simulink model "RST_CU_ESTIMATOR"  (R2018a)
settings: Solver=VariableStepAuto  StartTime=0.0  StopTime=100  RelTol=1e-3
values from neighbouring files (symbols this model uses):
  a22 = -2*beta*(c+f10)/numitor    (= -0.0723201373103)    [Proiect_script_IRA2.m]    (also in decupalre.m; trying.m)
  a23 = -M*g*L*f10/numitor    (= -43.7694067093)    [Proiect_script_IRA2.m]    (also in decupalre.m; trying.m)
  a24 = 2*beta*(c+f10)/numitor    (= 0.0723201373103)    [Proiect_script_IRA2.m]    (also in decupalre.m; trying.m)
  a42 = 2*beta*(d+f10)/numitor    (= 0.0279773616358)    [Proiect_script_IRA2.m]    (also in decupalre.m; trying.m)
  a43 = d*M*g*L/numitor    (= 43.7747367103)    [Proiect_script_IRA2.m]    (also in decupalre.m; trying.m)
  a44 = 2*beta*(d+f10)/numitor    (= 0.0279773616358)    [Proiect_script_IRA2.m]    (also in decupalre.m = -0.0279773616358; trying.m = -0.0279773616358)
  a66 = ((-W*W*beta)/(2*R*R))/(m*W*W/2+W*W/(2*R*R)*(Jw+Jm)+Jphi)    (= -0.112438053457)    [Proiect_script_IRA2.m]    (also in decupalre.m; trying.m)
  b21 = alfa*(c+f10)/numitor    (= 1.04508868945)    [Proiect_script_IRA2.m]    (also in decupalre.m; trying.m)
  b22 = alfa*(c+f10)/numitor    (= 1.04508868945)    [Proiect_script_IRA2.m]    (also in decupalre.m; trying.m)
  b41 = -alfa*(d+f10)/numitor    (= -0.404297133465)    [Proiect_script_IRA2.m]    (also in decupalre.m; trying.m)
  b42 = -alfa*(d+f10)/numitor    (= -0.404297133465)    [Proiect_script_IRA2.m]    (also in decupalre.m; trying.m)
  b61 = ((-W*alfa)/(2*R))/(m*W*W/2+W*W/(2*R*R)*(Jw+Jm)+Jphi)    (= -0.609310260785)    [Proiect_script_IRA2.m]    (also in decupalre.m; trying.m)
  b62 = ((-W*alfa)/(2*R))/(m*W*W/2+W*W/(2*R*R)*(Jw+Jm)+Jphi)    (= -0.609310260785)    [Proiect_script_IRA2.m]    (also in decupalre.m; trying.m)
  F1 = inv(C1/(-A0)*B1)    [Proiect_script_IRA2.m]    (also in decupalre.m; trying.m)
  k1 = acker(A1,B1,[-50 -50 -50 -50])    [Proiect_script_IRA2.m]    (also in decupalre.m = acker(A1,B1,[-10 -10 -10 -10]); trying.m = acker(A1,B1,[-2 -2 -2 -2]))
  k3 = acker(A2,B2,[-50 -50])    [Proiect_script_IRA2.m]    (also in decupalre.m = acker(A2,B2,[-1 -1]); trying.m = acker(A2,B2,[-0.01 -0.01]))
  Lt1 = acker(A1',C1',[-1000 -1000 -1000 -1000])    [Proiect_script_IRA2.m]    (also in trying.m)
  Lt3 = acker(A2',C2',[-1000 -1000])    [Proiect_script_IRA2.m]    (also in trying.m)
settings Model: Creator=Andrei  LastModifiedBy=Andrei

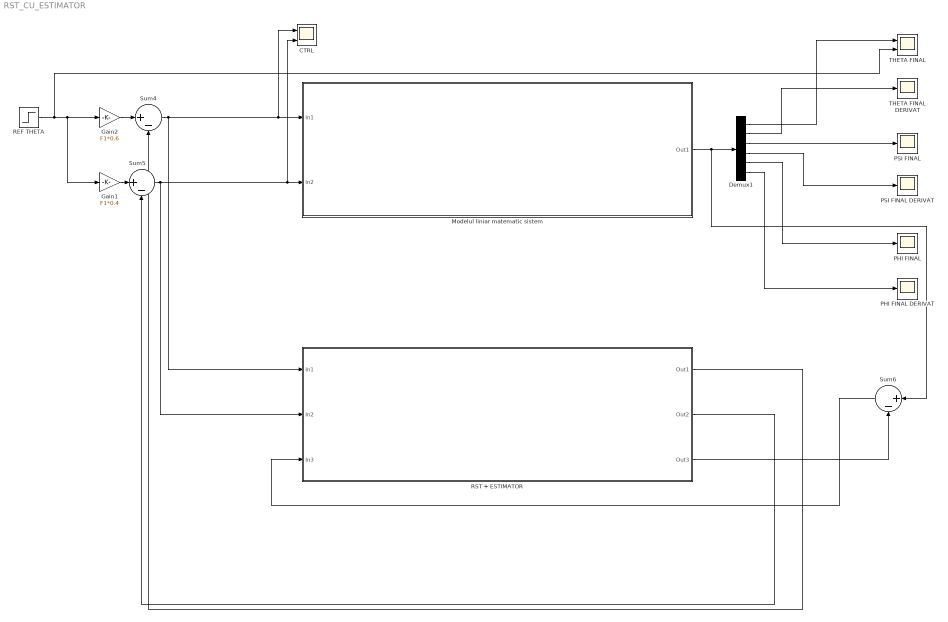
== system RST_CU_ESTIMATOR ==
  "CTRL " : Scope  NumInputPorts=2
  Demux1 : Demux  Outputs=6
  Gain1 : Gain  Gain=F1*0.4
  Gain2 : Gain  Gain=F1*0.6
  Modelul liniar matematic sistem : Subsystem
  PHI FINAL : Scope
  "PHI FINAL DERIVAT " : Scope
  PSI FINAL : Scope
  "PSI FINAL DERIVAT " : Scope
  "REF THETA " : Step  SampleTime=0
  "RST + ESTIMATOR " : Subsystem
  Sum4 : Sum  Inputs=|+-
  Sum5 : Sum  Inputs=|+-
  Sum6 : Sum  Inputs=|+-
  THETA FINAL : Scope  NumInputPorts=2
  "THETA FINAL DERIVAT " : Scope
  wires:
  Demux1/4 -> "PSI FINAL DERIVAT "/1
  "RST + ESTIMATOR "/1(Out1) -> Sum4/2
  Demux1/3 -> PSI FINAL/1
  Demux1/6 -> "PHI FINAL DERIVAT "/1
  Demux1/5 -> PHI FINAL/1
  Sum5/1 -> "RST + ESTIMATOR "/2(In2), Modelul liniar matematic sistem/2(In2), "CTRL "/2
  "RST + ESTIMATOR "/3(Out3) -> Sum6/2
  Demux1/1 -> THETA FINAL/1
  Gain2/1 -> Sum4/1
  Sum4/1 -> "RST + ESTIMATOR "/1(In1), Modelul liniar matematic sistem/1(In1), "CTRL "/1
  "RST + ESTIMATOR "/2(Out2) -> Sum5/2
  Modelul liniar matematic sistem/1(Out1) -> Demux1/1, Sum6/1
  Demux1/2 -> "THETA FINAL DERIVAT "/1
  Sum6/1 -> "RST + ESTIMATOR "/3(In3)
  "REF THETA "/1 -> THETA FINAL/2, Gain1/1, Gain2/1
  Gain1/1 -> Sum5/1

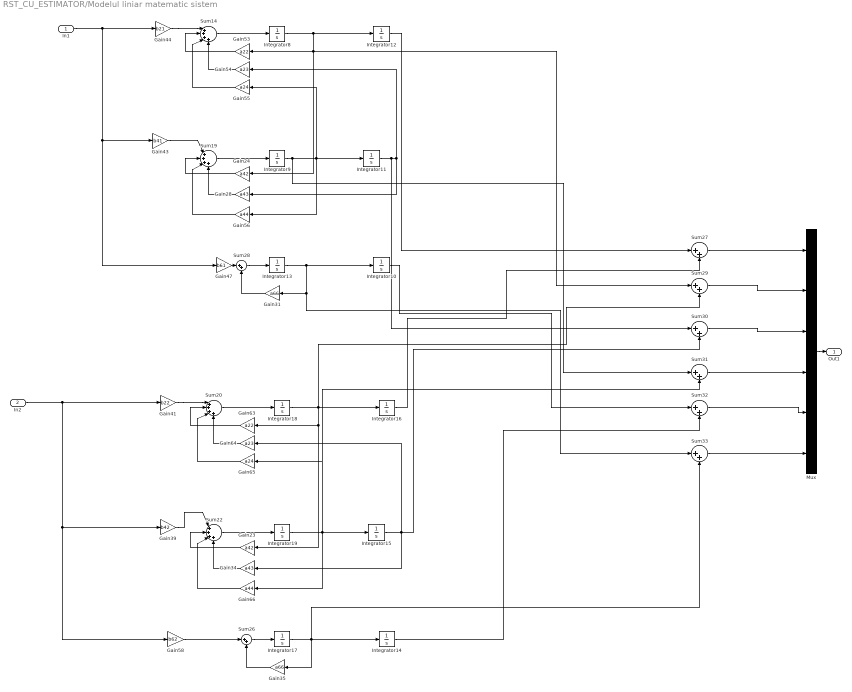
== system RST_CU_ESTIMATOR/Modelul liniar matematic sistem ==
  In1 : Inport
  In2 : Inport  Port=2
  Gain23 : Gain  Gain=a42
  Gain24 : Gain  Gain=a42
  Gain28 : Gain  Gain=a43
  Gain31 : Gain  Gain=a66
  Gain34 : Gain  Gain=a43
  Gain35 : Gain  Gain=a66
  Gain39 : Gain  Gain=b42
  Gain41 : Gain  Gain=b22
  Gain43 : Gain  Gain=b41
  Gain44 : Gain  Gain=b21
  Gain47 : Gain  Gain=b61
  Gain53 : Gain  Gain=a22
  Gain54 : Gain  Gain=a23
  Gain55 : Gain  Gain=a24
  Gain56 : Gain  Gain=a44
  Gain58 : Gain  Gain=b62
  Gain63 : Gain  Gain=a22
  Gain64 : Gain  Gain=a23
  Gain65 : Gain  Gain=a24
  Gain66 : Gain  Gain=a44
  Integrator{8..19} (12 alike) : Integrator
  Mux : Mux  Inputs=6
  Sum{14,19..20,22} (4 alike) : Sum  Inputs=|++++
  Sum{26..33} (8 alike) : Sum  Inputs=|++
  Out1 : Outport
  wires:
  In2/1 -> Gain41/1, Gain58/1, Gain39/1
  In1/1 -> Gain44/1, Gain43/1, Gain47/1
  Gain58/1 -> Sum26/1
  Sum26/1 -> Integrator17/1
  Integrator10/1 -> Sum32/1
  Gain56/1 -> Sum19/3
  Gain65/1 -> Sum20/3
  Integrator12/1 -> Sum27/1
  Sum29/1 -> Mux/2
  Sum31/1 -> Mux/4
  Gain23/1 -> Sum22/2
  Gain63/1 -> Sum20/2
  Gain35/1 -> Sum26/2
  Gain43/1 -> Sum19/1
  Sum28/1 -> Integrator13/1
  Gain47/1 -> Sum28/1
  Gain28/1 -> Sum19/4
  Integrator15/1 -> Gain34/1, Gain64/1, Sum30/2
  Integrator16/1 -> Sum27/2
  Sum27/1 -> Mux/1
  Gain34/1 -> Sum22/4
  Gain41/1 -> Sum20/1
  Integrator13/1 -> Integrator10/1, Gain31/1, Sum33/1
  Integrator11/1 -> Gain28/1, Gain54/1, Sum30/1
  Gain54/1 -> Sum14/4
  Integrator14/1 -> Sum32/2
  Gain64/1 -> Sum20/4
  Sum33/1 -> Mux/6
  Sum19/1 -> Integrator9/1
  Gain53/1 -> Sum14/2
  Gain24/1 -> Sum19/2
  Integrator18/1 -> Integrator16/1, Gain63/1, Gain23/1, Sum29/2
  Mux/1 -> Out1/1
  Sum22/1 -> Integrator19/1
  Integrator8/1 -> Integrator12/1, Gain53/1, Sum29/1, Gain24/1
  Gain44/1 -> Sum14/1
  Sum30/1 -> Mux/3
  Integrator17/1 -> Sum33/2, Integrator14/1, Gain35/1
  Sum14/1 -> Integrator8/1
  Sum20/1 -> Integrator18/1
  Gain55/1 -> Sum14/3
  Gain39/1 -> Sum22/1
  Sum32/1 -> Mux/5
  Integrator19/1 -> Gain65/1, Gain66/1, Sum31/2, Integrator15/1
  Gain66/1 -> Sum22/3
  Gain31/1 -> Sum28/2
  Integrator9/1 -> Integrator11/1, Gain55/1, Gain56/1, Sum31/1

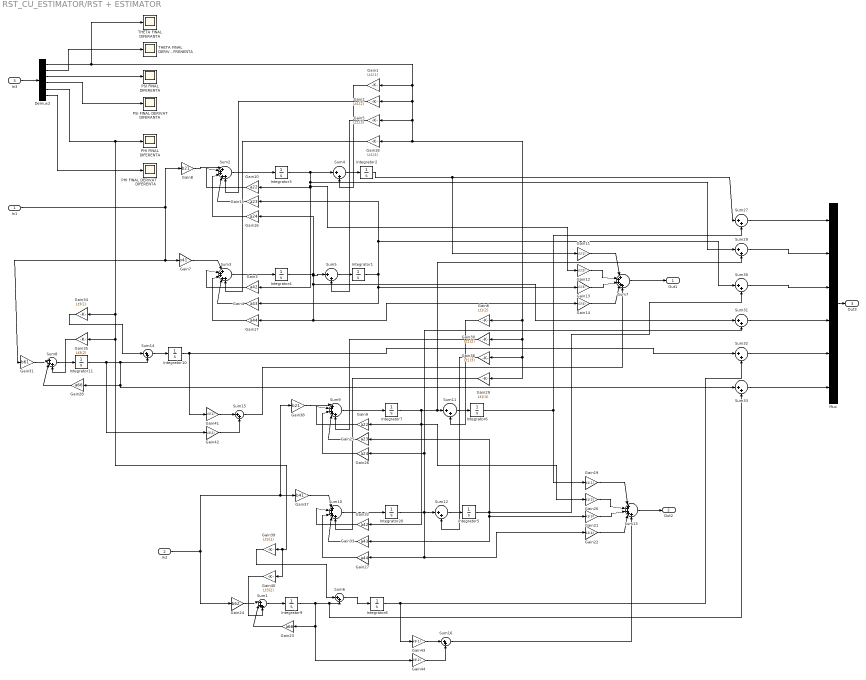
== system RST_CU_ESTIMATOR/RST + ESTIMATOR  ==
  In1 : Inport
  In2 : Inport  Port=2
  In3 : Inport  Port=3
  Demux2 : Demux  Outputs=6
  Gain1 : Gain  Gain=Lt1(1)
  Gain10 : Gain  Gain=a22
  Gain11 : Gain  Gain=k1(1)
  Gain12 : Gain  Gain=k1(2)
  Gain13 : Gain  Gain=k1(3)
  Gain14 : Gain  Gain=k1(4)
  Gain15 : Gain  Gain=a23
  Gain16 : Gain  Gain=a24
  Gain17 : Gain  Gain=a44
  Gain18 : Gain  Gain=Lt1(4)
  Gain19 : Gain  Gain=k1(1)
  Gain2 : Gain  Gain=Lt1(2)
  Gain20 : Gain  Gain=k1(2)
  Gain21 : Gain  Gain=k1(3)
  Gain22 : Gain  Gain=k1(4)
  Gain23 : Gain  Gain=a66
  Gain24 : Gain  Gain=b62
  Gain25 : Gain  Gain=a23
  Gain26 : Gain  Gain=a24
  Gain27 : Gain  Gain=a44
  Gain28 : Gain  Gain=a66
  Gain29 : Gain  Gain=Lt1(4)
  Gain3 : Gain  Gain=a42
  Gain30 : Gain  Gain=Lt1(2)
  Gain31 : Gain  Gain=b61
  Gain32 : Gain  Gain=a42
  Gain33 : Gain  Gain=a43
  Gain34 : Gain  Gain=Lt3(1)
  Gain35 : Gain  Gain=Lt3(2)
  Gain36 : Gain  Gain=Lt1(3)
  Gain37 : Gain  Gain=b41
  Gain38 : Gain  Gain=b21
  Gain39 : Gain  Gain=Lt3(1)
  Gain4 : Gain  Gain=a43
  Gain40 : Gain  Gain=Lt3(2)
  Gain41 : Gain  Gain=k3(1)
  Gain42 : Gain  Gain=k3(2)
  Gain43 : Gain  Gain=k3(1)
  Gain44 : Gain  Gain=k3(2)
  Gain5 : Gain  Gain=Lt1(3)
  Gain6 : Gain  Gain=Lt1(2)
  Gain7 : Gain  Gain=b41
  Gain8 : Gain  Gain=b21
  Gain9 : Gain  Gain=a22
  Integrator{1..11,20} (12 alike) : Integrator
  Mux : Mux  Inputs=6
  PHI FINAL DERIVAT DIFERENTA : Scope
  PHI FINAL DIFERENTA : Scope
  PSI FINAL DERIVAT DIFERANTA : Scope
  PSI FINAL DIFERENTA : Scope
  Sum1 : Sum  Inputs=|+++
  Sum{2..3,7,9..10,13} (6 alike) : Sum  Inputs=|+++++
  Sum{4..6,11..12,14..16,27,29..33} (14 alike) : Sum  Inputs=|++
  Sum8 : Sum  Inputs=|+++
  THETA FINAL DERIVAT DIFRENENTA : Scope
  THETA FINAL DIFERANTA : Scope
  Out1 : Outport
  Out2 : Outport  Port=2
  Out3 : Outport  Port=3
  wires:
  In3/1 -> Demux2/1
  Demux2/4 -> PSI FINAL DERIVAT DIFERANTA/1
  Demux2/6 -> PHI FINAL DERIVAT DIFERENTA/1
  Demux2/3 -> PSI FINAL DIFERENTA/1
  Demux2/5 -> PHI FINAL DIFERENTA/1, Gain34/1, Gain35/1, Gain39/1, Gain40/1
  Demux2/2 -> THETA FINAL DERIVAT DIFRENENTA/1
  Gain43/1 -> Sum16/1
  Gain44/1 -> Sum16/2
  Gain42/1 -> Sum15/2
  Gain41/1 -> Sum15/1
  Integrator8/1 -> Sum32/2, Gain43/1
  Integrator10/1 -> Sum32/1, Gain41/1
  Gain35/1 -> Sum8/3
  Gain34/1 -> Sum14/1
  Gain40/1 -> Sum1/3
  Gain39/1 -> Sum6/1
  Gain31/1 -> Sum8/1
  Sum14/1 -> Integrator10/1
  Gain28/1 -> Sum8/2
  Sum8/1 -> Integrator11/1
  Integrator11/1 -> Gain28/1, Sum33/1, Sum14/2, Gain42/1
  Sum6/1 -> Integrator8/1
  Integrator9/1 -> Gain23/1, Gain44/1, Sum33/2, Sum6/2
  Gain23/1 -> Sum1/2
  Gain24/1 -> Sum1/1
  Sum1/1 -> Integrator9/1
  In1/1 -> Gain8/1, Gain7/1, Gain31/1
  Mux/1 -> Out3/1
  Sum33/1 -> Mux/6
  Sum29/1 -> Mux/2
  Sum32/1 -> Mux/5
  Sum27/1 -> Mux/1
  Sum31/1 -> Mux/4
  Sum30/1 -> Mux/3
  In2/1 -> Gain24/1, Gain37/1, Gain38/1
  Gain6/1 -> Sum11/2
  Gain10/1 -> Sum2/2
  Gain7/1 -> Sum3/1
  Gain27/1 -> Sum10/3
  Integrator1/1 -> Gain13/1, Gain4/1, Sum30/1, Gain15/1
  Gain15/1 -> Sum2/4
  Sum2/1 -> Integrator3/1
  Gain1/1 -> Sum4/2
  Gain17/1 -> Sum3/3
  Gain16/1 -> Sum2/3
  Gain18/1 -> Sum3/5
  Gain11/1 -> Sum7/1
  Integrator4/1 -> Gain16/1, Sum5/1, Gain17/1, Gain14/1, Sum31/1
  Gain12/1 -> Sum7/2
  Gain26/1 -> Sum9/3
  Sum4/1 -> Integrator2/1
  Gain4/1 -> Sum3/4
  Gain13/1 -> Sum7/3
  Integrator2/1 -> Sum27/1, Gain11/1
  Gain14/1 -> Sum7/4
  Gain2/1 -> Sum2/5
  Gain3/1 -> Sum3/2
  Gain5/1 -> Sum5/2
  Sum5/1 -> Integrator1/1
  Integrator3/1 -> Sum4/1, Sum29/1, Gain10/1, Gain3/1, Gain12/1
  Sum3/1 -> Integrator4/1
  Gain8/1 -> Sum2/1
  Gain29/1 -> Sum10/5
  Gain21/1 -> Sum13/3
  Sum11/1 -> Integrator6/1
  Gain33/1 -> Sum10/4
  Gain20/1 -> Sum13/2
  Gain19/1 -> Sum13/1
  Integrator20/1 -> Sum12/1, Gain27/1, Gain22/1, Sum31/2, Gain26/1
  Gain36/1 -> Sum12/2
  Gain32/1 -> Sum10/2
  Gain30/1 -> Sum9/5
  Gain22/1 -> Sum13/4
  Integrator6/1 -> Sum27/2, Gain19/1
  Demux2/1 -> THETA FINAL DIFERANTA/1, Gain1/1, Gain2/1, Gain5/1, Gain18/1, Gain6/1, Gain30/1, Gain36/1, Gain29/1
  Sum7/1 -> Out1/1
  Gain37/1 -> Sum10/1
  Gain25/1 -> Sum9/4
  Integrator7/1 -> Gain9/1, Gain32/1, Gain20/1, Sum29/2, Sum11/1
  Sum12/1 -> Integrator5/1
  Sum10/1 -> Integrator20/1
  Gain38/1 -> Sum9/1
  Gain9/1 -> Sum9/2
  Sum13/1 -> Out2/1
  Sum9/1 -> Integrator7/1
  Integrator5/1 -> Sum30/2, Gain25/1, Gain21/1, Gain33/1
  Sum15/1 -> Sum7/5
  Sum16/1 -> Sum13/5
